simulink model "APF_CTL_VIS_Obs_2023a"  (R2023a)
settings: Solver=ode4  StartTime=0.0  StopTime=tsim  FixedStep=baseRate  RelTol=1e-6  AbsTol=1e-6
values from neighbouring files (symbols this model uses):
  A = [0 0 0 1 0 0 ... (first row only)    [CTL_NEW.m]    (also in UKF_SPOT.m = [1 0 0 dt 0 0)
  a = 25.028    [CTL_NEW.m]
  a1 = shape(1)    [Cardioid.m]    (also in Run_Initializer.m = 0.3)
  a2 = shape(2)    [Cardioid.m]    (also in Run_Initializer.m = 0.3)
  a3 = shape(3)    [Cardioid.m]    (also in Run_Initializer.m = 0.4)
  adadelta_epsilon = 1e-5    (= 1e-05)    [Run_Initializer.m]
  adadelta_gamma = 0.37    [Run_Initializer.m]
  adagrad_epsilon = 1e-8    (= 1e-08)    [Run_Initializer.m]
  adagrad_eta = 0.18    [Run_Initializer.m]
  adam_beta_1 = 0.99    [Run_Initializer.m]
  adam_beta_2 = 0.999    [Run_Initializer.m]
  adam_epsilon = 1e-2    (= 0.01)    [Run_Initializer.m]
  adam_eta = 0.0163    [Run_Initializer.m]
  adamax_beta_1 = 0.5    [Run_Initializer.m]
  adamax_beta_2 = 0.999    [Run_Initializer.m]
  adamax_eta = 0.014    [Run_Initializer.m]
  alpha_Black = 0.9    [UKF_SPOT.m]
  alpha_Blue = 0.9    [UKF_SPOT.m]
  Att_Mode = 0    [Run_Initializer.m]
  b1 = shape(4)    [Cardioid.m]    (also in Run_Initializer.m = 0.175)
  b2 = shape(5)    [Cardioid.m]    (also in Run_Initializer.m = 0.175)
  beta_Black = 2    [UKF_SPOT.m]
  beta_Blue = 20    [UKF_SPOT.m]
  Binv = inv(B)    [Run_Initializer.m]
  BLACK_end = [2, 1.4, deg2rad(368)]    [Run_Initializer.m]
  BLACK_ini = [2, 1.4, deg2rad(188), 0, 0, deg2rad(1.5)]    [Run_Initializer.m]
  BLUE_end = [1.3, 1.25, deg2rad(90)]    [Run_Initializer.m]
  BLUE_ini = [1.3, 1.25, deg2rad(270), 0, 0, deg2rad(-1.5)]    [Run_Initializer.m]
  drop_states_BLACK = BLACK_ini(1:3)    [Run_Initializer.m]
  drop_states_BLUE = BLUE_ini(1:3)    [Run_Initializer.m]
  drop_states_RED = RED_ini(1:3)    [Run_Initializer.m]
  dt = 0.01    [UKF_SPOT.m]
  end_time_black = 300    [Run_Initializer.m]
  end_time_blue = 300    [Run_Initializer.m]
  F_max = 0.22    [CTL_NEW.m]
  Gamma1_el = 0.12    [Run_Initializer.m]
  Gamma1_sh = 0.005    [Run_Initializer.m]
  Gamma1_wr = 0.025    [Run_Initializer.m]
  Gamma2_el = 5    [Run_Initializer.m]
  Gamma2_sh = 5    [Run_Initializer.m]
  Gamma2_wr = 5    [Run_Initializer.m]
  Gamma3_el = 10    [Run_Initializer.m]
  Gamma3_sh = 40    [Run_Initializer.m]
  Gamma3_wr = 40    [Run_Initializer.m]
  Gamma4_el = 0.039    [Run_Initializer.m]
  Gamma4_sh = 0.015    [Run_Initializer.m]
  Gamma4_wr = 0.029    [Run_Initializer.m]
  Gamma5_el = 800    [Run_Initializer.m]
  Gamma5_sh = 800    [Run_Initializer.m]
  Gamma5_wr = 800    [Run_Initializer.m]
  Gamma6_el = 0.000001    (= 1e-06)    [Run_Initializer.m]
  Gamma6_sh = 0.005    [Run_Initializer.m]
  Gamma6_wr = 0.02    [Run_Initializer.m]
  H = [1 0 0 0 0 0 ... (first row only)    [UKF_SPOT.m]
  home_states_BLACK = BLACK_ini(1:3)    [Run_Initializer.m]
  home_states_BLUE = BLUE_ini(1:3)    [Run_Initializer.m]
  home_states_RED = RED_ini(1:3)    [Run_Initializer.m]
  Hz = 0.01    [CTL_NEW.m]
  init_states_BLACK = BLACK_ini(1:3)    [Run_Initializer.m]
  init_states_BLUE = BLUE_ini(1:3)    [Run_Initializer.m]
  init_states_RED = RED_ini(1:3)    [Run_Initializer.m]
  J = IRED    [CTL_NEW.m]    (also in UKF_SPOT.m = 0.20184)
  k = lqr(A,B1,Q,R)    [CTL_NEW.m]
  k_1_0 = k(1,1)    [CTL_NEW.m]
  k_1_t_0 = k(3,3)    [CTL_NEW.m]
  k_2_0 = k(1,4)    [CTL_NEW.m]
  k_2_t_0 = k(3,6)    [CTL_NEW.m]
  K_a = diag([2 2 3.5])    [Run_Initializer.m]
  ka = 1    [Run_Initializer.m]
  Kd_elarm = 0.8    [Run_Initializer.m]
  Kd_sharm = 1.0    (= 1)    [Run_Initializer.m]
  Kd_t = 9.5    [CTL_NEW.m]    (also in Run_Initializer.m)
  Kd_wrarm = 0.6    [Run_Initializer.m]
  Kd_x = 28    [CTL_NEW.m]    (also in Run_Initializer.m)
  Kd_y = Kd_x    (= 28)    [CTL_NEW.m]    (also in Run_Initializer.m)
  Kp_elarm = 1.2    [Run_Initializer.m]
  Kp_sharm = 1.5    [Run_Initializer.m]
  Kp_t = 1    [CTL_NEW.m]    (also in Run_Initializer.m)
  Kp_wrarm = 2    [Run_Initializer.m]
  Kp_x = 3.5    [CTL_NEW.m]    (also in Run_Initializer.m)
  Kp_y = Kp_x    (= 3.5)    [CTL_NEW.m]    (also in Run_Initializer.m)
  kr = 2    [Run_Initializer.m]
  lambda1 = 0.4    [CTL_NEW.m]
  lambda12 = 0.4    [CTL_NEW.m]
  lambda12_t = 0.05    [CTL_NEW.m]
  lambda1_t = 0.05    [CTL_NEW.m]
  lambda2 = 0.4    [CTL_NEW.m]
  lambda2_t = 0.05    [CTL_NEW.m]
  lamda_Black = (alpha_Black^2)*(N + kappa_Black) - N    (= 15.06)    [UKF_SPOT.m]
  lamda_Blue = (alpha_Blue^2)*(N + kappa_Blue) - N    (= 6.96)    [UKF_SPOT.m]
  m = mRED    [CTL_NEW.m]    (also in UKF_SPOT.m = 11.21)
  method = 1    [UKF_SPOT.m]
  Method = 8    [Run_Initializer.m]
  momentum_eta = 0.7    [Run_Initializer.m]
  momentum_gamma = 0.7    [Run_Initializer.m]
  nesterov_eta = 0.6    [Run_Initializer.m]
  nesterov_gamma = 0.3    [Run_Initializer.m]
  Nmat = diag([1 1 1])    [Run_Initializer.m]
  p = 0.4    [CTL_NEW.m]
  P_b = diag([45 45 0])    [Run_Initializer.m]
  P_IC_Black = 0.2*eye(6)    [UKF_SPOT.m]
  P_IC_Blue = 0.2*eye(6)    [UKF_SPOT.m]
  p_t = 0.05    [CTL_NEW.m]
  psi = 1    [Run_Initializer.m]
  PWMFreq = 5    [Run_Initializer.m]
  Q = [w 0 0 0 0 0 ... (first row only)    [CTL_NEW.m]
  Q_a = diag([5, 5, 0])    [Run_Initializer.m]
  Q_b = diag([0.0125, 0.0125, 0.05])    [Run_Initializer.m]
  Q_Black = [0.0000005 0 0 0 0 0 ... (first row only)    [UKF_SPOT.m]
  Q_Blue = [0.000075 0 0 0 0 0 ... (first row only)    [UKF_SPOT.m]
  R = [r 0 0 ... (first row only)    [CTL_NEW.m]
  R_Black = [variance 0 0 ... (first row only)    [UKF_SPOT.m]
  R_Blue = [variance 0 0 ... (first row only)    [UKF_SPOT.m]
  r_hold = 0.427    [Run_Initializer.m]
  r_off = 0.165    [Run_Initializer.m]
  RED_ini = [2.7, 0.4, deg2rad(135+360), 0, 0, 0]    [Run_Initializer.m]
  Red_Rate = 0.025    [CTL_NEW.m]
  RMSprop_epsilon = 1e-8    (= 1e-08)    [Run_Initializer.m]
  RMSprop_eta = 0.025    [Run_Initializer.m]
  RMSprop_gamma = 0.9    [Run_Initializer.m]
  ... (+11 more)
undefined symbols (not defined in the file or in its folder): alpha, alpha_m, alphap, alphat, Am, b, b0, b3, baseRate, beta, Bm, c, Cm, d, DiscIntNeverNeededParam, Dm, drop_states_ARM, epsilon, F_Black_X_nominal, F_Black_Y_nominal, F_Blue_X_nominal, F_Blue_Y_nominal, F_red_X_nominal, F_red_Y_nominal, F_thrusters_BLACK, F_thrusters_BLUE, F_thrusters_RED, IBLACK, IBLUE, IDIST, IEE, IPROX, IRED, K, k1, k1t, k2, k2t, K_t, Kd_tb, Kd_tblue, Kd_tr, Kd_xb, Kd_xblue, Kd_xr, Kd_yb, Kd_yblue, Kd_yr, Kp_tb, Kp_tblue, Kp_tr, Kp_xb, Kp_xblue, Kp_xr, Kp_yb, Kp_yblue, Kp_yr, lamda ... (+34)
libraries: nvidiaSharedBlocks x10, MainLibrary x4, dspsigops x4, simulink x2, etargetslib x1
(part 15 of 15)

== matlab function APF_CTL_VIS_Obs_2023a/Phase #3: Experiment/Change RED Behavior/Sub-Phase #4/GDC/APF/GDC/Subsystem1/AdaDelta/MATLAB Function1 ==
  data: state_red input size=6; path output size=3; Eg output size=3; phi_tot_grad input size=3; Eg_old input size=3; Etheta_old input size=3; Etheta output size=3; adadelta_gamma parameter size=1; adadelta_epsilon parameter size=1
function [path, Eg, Etheta] = AdaDel(state_red, phi_tot_grad,Eg_old, Etheta_old, adadelta_gamma, adadelta_epsilon)

Eg = adadelta_gamma.*Eg_old + (1 - adadelta_gamma).*((phi_tot_grad).^2);
del_theta = (sqrt(Etheta_old + adadelta_epsilon)./sqrt(Eg + adadelta_epsilon)).*phi_tot_grad;
Etheta = adadelta_gamma.*Etheta_old + (1 - adadelta_gamma).*((del_theta).^2);

path = state_red(1:3) - del_theta;

== matlab function APF_CTL_VIS_Obs_2023a/Phase #3: Experiment/Change RED Behavior/Sub-Phase #4/GDC/APF/GDC/Subsystem1/AdaGrad/MATLAB Function1 ==
  data: state_red input; path output; phi_tot_grad input; Gt_old input; adagrad_eta parameter; Gt output; adagrad_epsilon parameter
function [path, Gt] = AdaGrad(state_red, phi_tot_grad, Gt_old,adagrad_eta, adagrad_epsilon)

Gt = Gt_old + phi_tot_grad.^2;

n = adagrad_eta./sqrt(Gt + adagrad_epsilon);

path = state_red(1:3) - n.*phi_tot_grad;

== matlab function APF_CTL_VIS_Obs_2023a/Phase #3: Experiment/Change RED Behavior/Sub-Phase #4/GDC/APF/GDC/Subsystem1/Gradient Descent/Batch ==
  data: state_red input; path output; phi_tot_grad input; batch_eta parameter
function path = gradientdescent(state_red, phi_tot_grad, batch_eta)

%Batch Gradient Descent
path = [state_red(1); state_red(2); state_red(3)] - batch_eta.*phi_tot_grad;

== matlab function APF_CTL_VIS_Obs_2023a/Phase #3: Experiment/Change RED Behavior/Sub-Phase #4/GDC/APF/GDC/Subsystem1/AdaMax/MATLAB Function1 ==
  data: state_red input; path output; phi_tot_grad input; m_old input; m output; u_old input; time input; u_t output; adamax_beta_1 parameter; adamax_beta_2 parameter; adamax_eta parameter
function [path, m, u_t] = AdaMax(state_red, phi_tot_grad,m_old, u_old, time, adamax_beta_1, adamax_beta_2, adamax_eta)

t = time/0.1;
m = adamax_beta_1.*m_old + (1 - adamax_beta_1).*phi_tot_grad;
%v = adamax_beta_2.*v_old + (1 - adamax_beta_2).*norm(phi_tot_grad,"inf");

m_h = m./(1 - (adamax_beta_1)^(t + 1));
u_t = max(adamax_beta_2.*u_old, abs(phi_tot_grad));

path = state_red(1:3) - (adamax_eta./u_t).*m_h;

== matlab function APF_CTL_VIS_Obs_2023a/Phase #4: Return Home/Change BLACK Behavior/Hough Control/MATLAB Function2 ==
  data: Oy output; z input; Ox output
function [Oy, Ox]   = C3( z )
%C3 gives the rotation matrix about the z-axis for an angle 'z'
%   z - the angle about the z-axis which you rotate
%   A - the rotation matrix

Ox = [cos(z) sin(z); -sin(z) cos(z)]*[1;0];
Oy = [cos(z) sin(z); -sin(z) cos(z)]*[0;1];
end

== matlab function APF_CTL_VIS_Obs_2023a/Phase #4: Return Home/Change BLACK Behavior/Hough Control/MATLAB Function3 ==
  data: z input; Ox output
function Ox    = C3( z )
%C3 gives the rotation matrix about the z-axis for an angle 'z'
%   z - the angle about the z-axis which you rotate
%   A - the rotation matrix

Ox = [cos(z) sin(z); -sin(z) cos(z)]*[1;0];
end

== matlab function APF_CTL_VIS_Obs_2023a/Phase #4: Return Home/Change BLACK Behavior/Hough Control/MATLAB Function4 ==
  data: Oy input; e_out output; e_in input
function e_out = fcn(Oy, e_in)

a = sign(Oy'*e_in);
e_out = -a*norm(e_in);

== matlab function APF_CTL_VIS_Obs_2023a/Phase #3: Experiment/Change RED Behavior/Sub-Phase #4/GDC/APF/GDC/Subsystem1/Adam/MATLAB Function1 ==
  data: state_red input; path output; phi_tot_grad input; m_old input; m output; v_old input; time input; v output; adam_beta_1 parameter; adam_beta_2 parameter; adam_eta parameter; adam_epsilon parameter
function [path, m, v] = Adam(state_red, phi_tot_grad,m_old, v_old, time, adam_beta_1, adam_beta_2, adam_eta, adam_epsilon)

m = adam_beta_1.*m_old + (1 - adam_beta_1).*phi_tot_grad;
v = adam_beta_2.*v_old + (1 - adam_beta_2).*(phi_tot_grad).^2;

m_h = m./(1 - (adam_beta_1)^(time/0.1 + 1));
v_h = v./(1 - (adam_beta_2)^(time/0.1 + 1));

path = state_red(1:3) - (adam_eta./(sqrt(v_h) + adam_epsilon)).*m_h;

== matlab function APF_CTL_VIS_Obs_2023a/Phase #3: Experiment/Change RED Behavior/Sub-Phase #4/GDC/APF/GDC/Subsystem1/Nesterov/MATLAB Function1 ==
  data: state_red input; path output; v_prev input; shape parameter; ka parameter; kr parameter; Q_a parameter; Q_b parameter; P_b parameter; r_hold parameter; Binv parameter; K_a parameter; psi parameter; sigma parameter; r_off parameter; Nmat parameter; nesterov_gamma parameter; v output; state_black input; state_blue input; nesterov_eta parameter; isBlue input
function [path, v] = nesterov(state_red, v_prev, shape, ka, kr, Q_a, Q_b, P_b, r_hold, Binv, K_a, psi, sigma, r_off, Nmat, nesterov_gamma, state_black, state_blue, nesterov_eta,isBlue)
%Nesterov Accelerated Gradient

state_red_est = state_red + nesterov_gamma.*[v_prev(1); v_prev(2); v_prev(3); 0; 0; 0];
[~,phi_tot_grad,~,~] = APF_func_Maybe_Obstacle(state_red_est,state_black,state_blue,shape,ka,kr,Q_a,Q_b,P_b,r_hold,Binv,K_a,psi,sigma,r_off,Nmat,isBlue); %calculates the gradient if 

v = -nesterov_gamma*v_prev-nesterov_eta.*phi_tot_grad;
path = [state_red(1); state_red(2); state_red(3)] + v;

== matlab function APF_CTL_VIS_Obs_2023a/Phase #3: Experiment/Change BLUE Behavior/Sub-Phase #1/BLUE_Rz Desired/Wrap/MATLAB Function ==
  data: u input; wrappedAngle output
function wrappedAngle = wrapAngle(u)

wrappedAngle = atan2(sin(u),cos(u));

end

== matlab function APF_CTL_VIS_Obs_2023a/Phase #3: Experiment/Change BLACK Behavior/Sub-Phase #4/Hough Control/MATLAB Function4 ==
  data: Oy input; e_out output; e_in input
function e_out = fcn(Oy, e_in)

a = sign(Oy'*e_in);
e_out = -a*norm(e_in);

== matlab function APF_CTL_VIS_Obs_2023a/Phase #4: Return Home/Change BLUE Behavior/Hough Control/MATLAB Function2 ==
  data: Oy output; z input; Ox output
function [Oy, Ox]   = C3( z )
%C3 gives the rotation matrix about the z-axis for an angle 'z'
%   z - the angle about the z-axis which you rotate
%   A - the rotation matrix

Ox = [cos(z) sin(z); -sin(z) cos(z)]*[1;0];
Oy = [cos(z) sin(z); -sin(z) cos(z)]*[0;1];
end

== matlab function APF_CTL_VIS_Obs_2023a/Phase #4: Return Home/Change BLUE Behavior/Hough Control/MATLAB Function3 ==
  data: z input; Ox output
function Ox    = C3( z )
%C3 gives the rotation matrix about the z-axis for an angle 'z'
%   z - the angle about the z-axis which you rotate
%   A - the rotation matrix

Ox = [cos(z) sin(z); -sin(z) cos(z)]*[1;0];
end

== matlab function APF_CTL_VIS_Obs_2023a/Phase #4: Return Home/Change BLUE Behavior/Hough Control/MATLAB Function4 ==
  data: Oy input; e_out output; e_in input
function e_out = fcn(Oy, e_in)

a = sign(Oy'*e_in);
e_out = -a*norm(e_in);

== matlab function APF_CTL_VIS_Obs_2023a/Phase #4: Return Home/Change RED Behavior/Hough Control/MATLAB Function2 ==
  data: Oy output; z input; Ox output
function [Oy, Ox]   = C3( z )
%C3 gives the rotation matrix about the z-axis for an angle 'z'
%   z - the angle about the z-axis which you rotate
%   A - the rotation matrix

Ox = [cos(z) sin(z); -sin(z) cos(z)]*[1;0];
Oy = [cos(z) sin(z); -sin(z) cos(z)]*[0;1];
end

== matlab function APF_CTL_VIS_Obs_2023a/Phase #4: Return Home/Change RED Behavior/Hough Control/MATLAB Function3 ==
  data: z input; Ox output
function Ox    = C3( z )
%C3 gives the rotation matrix about the z-axis for an angle 'z'
%   z - the angle about the z-axis which you rotate
%   A - the rotation matrix

Ox = [cos(z) sin(z); -sin(z) cos(z)]*[1;0];
end

== matlab function APF_CTL_VIS_Obs_2023a/Phase #4: Return Home/Change RED Behavior/Hough Control/MATLAB Function4 ==
  data: Oy input; e_out output; e_in input
function e_out = fcn(Oy, e_in)

a = sign(Oy'*e_in);
e_out = -a*norm(e_in);

== matlab function APF_CTL_VIS_Obs_2023a/Thruster Control Code/Change RED Behavior/Calculate Thruster ON//OFF/MATLAB Function ==
  data: H output; thruster_dist2CG_RED parameter; F_thrusters_RED parameter; theta_1 input; theta_2 input; theta_3 input; mRED parameter; mPROX parameter; mDIST parameter; mEE parameter; Phi parameter; b0 parameter; a1 parameter; b1 parameter; a2 parameter; b2 parameter; a3 parameter; b3 parameter
function H   = MakeHWithArm(thruster_dist2CG_RED,F_thrusters_RED, theta_1, theta_2, theta_3, mRED, mPROX, mDIST, mEE, Phi, b0, a1, b1, a2, b2, a3, b3)
    
    link1_com_x = b0*cos(Phi) + a1*cos(pi/2 + theta_1);
    link1_com_y = b0*sin(Phi) + a1*sin(pi/2 + theta_1);
    
    link2_com_x = link1_com_x + b1*cos(pi/2 + theta_1) + a2*cos(pi/2 + theta_1 + theta_2);
    link2_com_y = link1_com_y + b1*sin(pi/2 + theta_1) + a2*sin(pi/2 + theta_1 + theta_2);
    
    link3_com_x = link2_com_x + b2*cos(pi/2 + theta_1 + theta_2) + a3*cos(pi/2 + theta_1 + theta_2 + theta_3);
    link3_com_y = link2_com_y + b2*sin(pi/2 + theta_1 + theta_2) + a3*sin(pi/2 + theta_1 + theta_2 + theta_3);
    
    delta_com_due_to_arm_x = (mPROX*link1_com_x + mDIST*link2_com_x + mEE*link3_com_x)/(mRED + mPROX + mDIST + mEE)*1000; % [mm]
    delta_com_due_to_arm_y = (mPROX*link1_com_y + mDIST*link2_com_y + mEE*link3_com_y)/(mRED + mPROX + mDIST + mEE)*1000; % [mm]
    
    adjusted_thruster_dist2CG_RED = [thruster_dist2CG_RED(1)-delta_com_due_to_arm_y;
                                     thruster_dist2CG_RED(2)-delta_com_due_to_arm_y;
                                     thruster_dist2CG_RED(3)-delta_com_due_to_arm_x;
                                     thruster_dist2CG_RED(4)-delta_com_due_to_arm_x;
                                     thruster_dist2CG_RED(5)+delta_com_due_to_arm_y;
                                     thruster_dist2CG_RED(6)+delta_com_due_to_arm_y;
                                     thruster_dist2CG_RED(7)+delta_com_due_to_arm_x;
                                     thruster_dist2CG_RED(8)+delta_com_due_to_arm_x];
                                     
    
    
    Vec1 = [ -1
             -1
              0 
              0
              1
              1
              0
              0 ];
          
    Vec2 = [  0
              0
              1
              1
              0
              0
             -1
             -1 ];
         
    Vec3 = adjusted_thruster_dist2CG_RED./1000;
    
    Mat1 = [Vec1, Vec2, Vec3]';
    
    Mat2 = diag((F_thrusters_RED./2));
    
    H    = Mat1*Mat2;

end

== matlab function APF_CTL_VIS_Obs_2023a/Phase #3: Experiment/Change BLUE Behavior/Sub-Phase #2 /BLUE_Rz Desired/Wrap/MATLAB Function ==
  data: u input; wrappedAngle output
function wrappedAngle = wrapAngle(u)

wrappedAngle = atan2(sin(u),cos(u));

end

== matlab function APF_CTL_VIS_Obs_2023a/Thruster Control Code/Change BLACK Behavior/Calculate Thruster ON//OFF/MATLAB Function3 ==
  data: H output; thruster_dist2CG_BLACK parameter; F_Black_X_nominal parameter; thrust_decay_factor input; F_Black_Y_nominal parameter
function H   = MakeHWithDecay(thruster_dist2CG_BLACK,F_Black_X_nominal, thrust_decay_factor, F_Black_Y_nominal)


adjusted_thruster_dist2CG_BLACK = [thruster_dist2CG_BLACK(1);
                                 thruster_dist2CG_BLACK(2);
                                 thruster_dist2CG_BLACK(3);
                                 thruster_dist2CG_BLACK(4);
                                 thruster_dist2CG_BLACK(5);
                                 thruster_dist2CG_BLACK(6);
                                 thruster_dist2CG_BLACK(7);
                                 thruster_dist2CG_BLACK(8)];
                                 


Vec1 = [ -1
         -1
          0 
          0
          1
          1
          0
          0 ];
      
Vec2 = [  0
          0
          1
          1
          0
          0
         -1
         -1 ];
     
Vec3 = adjusted_thruster_dist2CG_BLACK./1000;

Mat1 = [Vec1, Vec2, Vec3]';

F_thrusters_BLACK = [F_Black_X_nominal*thrust_decay_factor; F_Black_X_nominal*thrust_decay_factor; F_Black_Y_nominal*thrust_decay_factor; F_Black_Y_nominal*thrust_decay_factor; F_Black_X_nominal*thrust_decay_factor; F_Black_X_nominal*thrust_decay_factor; F_Black_Y_nominal*thrust_decay_factor; F_Black_Y_nominal*thrust_decay_factor];

Mat2 = diag((F_thrusters_BLACK));

H    = Mat1*Mat2;

end

== matlab function APF_CTL_VIS_Obs_2023a/Thruster Control Code/Change RED Behavior/Calculate Thruster ON//OFF/MATLAB Function2 ==
  data: ThrustPer_Final output; ThrustPer input; PWMFreq parameter
function ThrustPer_Final  = ThrusterSat(ThrustPer, PWMFreq)

    ValveTime       = 0.007;
    TControl        = 1/PWMFreq;

    ThrustPer_Final = zeros(8,1);
    
    if max(ThrustPer) > 1
        ThrustPer_Sat = ThrustPer/max(ThrustPer);
    else
        ThrustPer_Sat = ThrustPer;
    end
    
    for i = 1:8
        if ThrustPer_Sat(i) > ValveTime/TControl 
            ThrustPer_Final(i) = ThrustPer_Sat(i);
        else
            ThrustPer_Final(i) = 0;
        end
    end


end

== matlab function APF_CTL_VIS_Obs_2023a/Thruster Control Code/Change RED Behavior/Calculate Thruster ON//OFF/Rotate Forces to Inertial/Create Rotation Matrix ==
  data: Rz input; C_Ib output
function C_Ib = RotateFrame(Rz)

C_bI = [  cos(Rz) sin(Rz)
         -sin(Rz) cos(Rz) ];

C_Ib = inv(C_bI);

end

== matlab function APF_CTL_VIS_Obs_2023a/Phase #3: Experiment/Change BLACK Behavior/Sub-Phase #2 /BLACK_Rz Desired/Wrap1/MATLAB Function ==
  data: u input; wrappedAngle output
function wrappedAngle = wrapAngle(u)

wrappedAngle = atan2(sin(u),cos(u));

end

== matlab function APF_CTL_VIS_Obs_2023a/Phase #3: Experiment/Change RED Behavior/Sub-Phase #1/MATLAB Function ==
  data: t input; x output; xLength parameter
function x = fcn(t, xLength)

x = 0.9*cos((0.03490659)*t) + xLength/2;

end

== matlab function APF_CTL_VIS_Obs_2023a/Phase #3: Experiment/Change RED Behavior/Sub-Phase #4/GDC/APF/GDC/Subsystem1/RMSProp/MATLAB Function1 ==
  data: state_red input; path output; phi_tot_grad input; Eg_old input; Eg output; RMSprop_eta parameter; RMSprop_gamma parameter; RMSprop_epsilon parameter
function [path, Eg] = RMSProp(state_red, phi_tot_grad, Eg_old, RMSprop_eta, RMSprop_gamma, RMSprop_epsilon)

Eg = RMSprop_gamma.*Eg_old + (1 - RMSprop_gamma).*((phi_tot_grad).^2);

n = RMSprop_eta./sqrt(Eg + RMSprop_epsilon);

path = state_red(1:3) - n.*phi_tot_grad;

== matlab function APF_CTL_VIS_Obs_2023a/Simulate Plant Dynamics/RED and ARM Dynamics/RED + ARM/RED + ARM Dynamics/Dynamics Model ==
  data: xdot output; x input; InertiaS input; CoriolisS input; u input; Gamma1_sh parameter; Gamma2_sh parameter; Gamma3_sh parameter; Gamma5_sh parameter; Gamma4_sh parameter; Gamma6_sh parameter; Gamma1_el parameter; Gamma2_el parameter; Gamma3_el parameter; Gamma5_el parameter; Gamma4_el parameter; Gamma6_el parameter; Gamma1_wr parameter; Gamma2_wr parameter; Gamma3_wr parameter; Gamma5_wr parameter; Gamma4_wr parameter; Gamma6_wr parameter
function xdot  = DynamicsModel(x, InertiaS, CoriolisS, u,...
    Gamma1_sh, Gamma2_sh, Gamma3_sh, Gamma5_sh, Gamma4_sh, Gamma6_sh,...
    Gamma1_el, Gamma2_el, Gamma3_el, Gamma5_el, Gamma4_el, Gamma6_el,...
    Gamma1_wr, Gamma2_wr, Gamma3_wr, Gamma5_wr, Gamma4_wr, Gamma6_wr)


    fqdot1 = Gamma1_sh*(tanh(Gamma2_sh*x(10)) - tanh(Gamma3_sh*x(10))) + Gamma4_sh*tanh(Gamma5_sh*x(10)) + Gamma6_sh*x(10);

    fqdot2 = Gamma1_el*(tanh(Gamma2_el*x(11)) - tanh(Gamma3_el*x(11))) + Gamma4_el*tanh(Gamma5_el*x(11)) + Gamma6_el*x(11);

    fqdot3 = Gamma1_wr*(tanh(Gamma2_wr*x(12)) - tanh(Gamma3_wr*x(12))) + Gamma4_wr*tanh(Gamma5_wr*x(12)) + Gamma6_wr*x(12);
    
    q_ddot = pinv(InertiaS)*(u - CoriolisS*x(7:12) - [0;0;0;fqdot1;fqdot2;fqdot3]);
    
    xdot   = [ x(7:12)
               q_ddot   ];
           
end

== matlab function APF_CTL_VIS_Obs_2023a/Phase #3: Experiment/Change BLUE Behavior/Sub-Phase #3 /BLUE_Rz Desired/Wrap/MATLAB Function ==
  data: u input; wrappedAngle output
function wrappedAngle = wrapAngle(u)

wrappedAngle = atan2(sin(u),cos(u));

end

== matlab function APF_CTL_VIS_Obs_2023a/Phase #3: Experiment/Change RED Behavior/Sub-Phase #4/CTL/If Action Subsystem/Homo/MATLAB Function2 ==
  data: q1 input; u output; k1 parameter; alphap parameter
function u = fcn(q1,k1, alphap)

u = k1*sign(q1)*(abs(q1)^(alphap/(2 - alphap)));

== matlab function APF_CTL_VIS_Obs_2023a/Phase #3: Experiment/Change RED Behavior/Sub-Phase #1/MATLAB Function1 ==
  data: t input; y output; yLength parameter
function y = fcn(t, yLength)

y = 0.85*sin((0.03490659)*t) + yLength/2;

end

== matlab function APF_CTL_VIS_Obs_2023a/Phase #3: Experiment/Change RED Behavior/Sub-Phase #2 /Hough Control/MATLAB Function2 ==
  data: Oy output; z input; Ox output
function [Oy, Ox]   = C3( z )
%C3 gives the rotation matrix about the z-axis for an angle 'z'
%   z - the angle about the z-axis which you rotate
%   A - the rotation matrix

Ox = [cos(z) sin(z); -sin(z) cos(z)]*[1;0];
Oy = [cos(z) sin(z); -sin(z) cos(z)]*[0;1];
end

== matlab function APF_CTL_VIS_Obs_2023a/Phase #3: Experiment/Change RED Behavior/Sub-Phase #2 /Hough Control/MATLAB Function3 ==
  data: z input; Ox output
function Ox    = C3( z )
%C3 gives the rotation matrix about the z-axis for an angle 'z'
%   z - the angle about the z-axis which you rotate
%   A - the rotation matrix

Ox = [cos(z) sin(z); -sin(z) cos(z)]*[1;0];
end

== matlab function APF_CTL_VIS_Obs_2023a/Phase #3: Experiment/Change BLACK Behavior/Sub-Phase #2 /Hough Control/MATLAB Function2 ==
  data: Oy output; z input; Ox output
function [Oy, Ox]   = C3( z )
%C3 gives the rotation matrix about the z-axis for an angle 'z'
%   z - the angle about the z-axis which you rotate
%   A - the rotation matrix

Ox = [cos(z) sin(z); -sin(z) cos(z)]*[1;0];
Oy = [cos(z) sin(z); -sin(z) cos(z)]*[0;1];
end

== matlab function APF_CTL_VIS_Obs_2023a/Phase #3: Experiment/Change RED Behavior/Sub-Phase #2 /Hough Control/MATLAB Function4 ==
  data: Oy input; e_out output; e_in input
function e_out = fcn(Oy, e_in)

a = sign(Oy'*e_in);
e_out = -a*norm(e_in);

== matlab function APF_CTL_VIS_Obs_2023a/Thruster Control Code/Change RED Behavior/Calculate Thruster ON//OFF/MATLAB Function3 ==
  data: H output; thruster_dist2CG_RED parameter; F_thrusters_RED parameter
function H = MakeH(thruster_dist2CG_RED,F_thrusters_RED)

Vec1 = [ -1
         -1
          0 
          0
          1
          1
          0
          0 ];
      
Vec2 = [  0
          0
          1
          1
          0
          0
         -1
         -1 ];
     
Vec3 = thruster_dist2CG_RED./1000;

Mat1 = [Vec1, Vec2, Vec3]';

Mat2 = diag((F_thrusters_RED));

H    = Mat1*Mat2;

end

== matlab function APF_CTL_VIS_Obs_2023a/Phase #3: Experiment/Change BLUE Behavior/Sub-Phase #4/BLUE_Rz Desired/Wrap/MATLAB Function ==
  data: u input; wrappedAngle output
function wrappedAngle = wrapAngle(u)

wrappedAngle = atan2(sin(u),cos(u));

end

== matlab function APF_CTL_VIS_Obs_2023a/Thruster Control Code/Change RED Behavior/Calculate Thruster ON//OFF/MATLAB Function4 ==
  data: H output; thruster_dist2CG_RED parameter; F_red_X_nominal parameter; theta_1 input; theta_2 input; theta_3 input; mRED parameter; thrust_decay_factor input; F_red_Y_nominal parameter; mPROX parameter; mDIST parameter; mEE parameter; Phi parameter; b0 parameter; a1 parameter; b1 parameter; a2 parameter; b2 parameter; a3 parameter; b3 parameter
function H   = MakeH(thruster_dist2CG_RED,F_red_X_nominal, theta_1, theta_2, theta_3, mRED, thrust_decay_factor, F_red_Y_nominal, mPROX, mDIST, mEE, Phi, b0, a1, b1, a2, b2, a3, b3)
    
    link1_com_x = b0*cos(Phi) + a1*cos(pi/2 + theta_1);
    link1_com_y = b0*sin(Phi) + a1*sin(pi/2 + theta_1);
    
    link2_com_x = link1_com_x + b1*cos(pi/2 + theta_1) + a2*cos(pi/2 + theta_1 + theta_2);
    link2_com_y = link1_com_y + b1*sin(pi/2 + theta_1) + a2*sin(pi/2 + theta_1 + theta_2);
    
    link3_com_x = link2_com_x + b2*cos(pi/2 + theta_1 + theta_2) + a3*cos(pi/2 + theta_1 + theta_2 + theta_3);
    link3_com_y = link2_com_y + b2*sin(pi/2 + theta_1 + theta_2) + a3*sin(pi/2 + theta_1 + theta_2 + theta_3);
    
    delta_com_due_to_arm_x = (mPROX*link1_com_x + mDIST*link2_com_x + mEE*link3_com_x)/(mRED + mPROX + mDIST + mEE)*1000; % [mm]
    delta_com_due_to_arm_y = (mPROX*link1_com_y + mDIST*link2_com_y + mEE*link3_com_y)/(mRED + mPROX + mDIST + mEE)*1000; % [mm]
    
    adjusted_thruster_dist2CG_RED = [thruster_dist2CG_RED(1)-delta_com_due_to_arm_y;
                                     thruster_dist2CG_RED(2)-delta_com_due_to_arm_y;
                                     thruster_dist2CG_RED(3)-delta_com_due_to_arm_x;
                                     thruster_dist2CG_RED(4)-delta_com_due_to_arm_x;
                                     thruster_dist2CG_RED(5)+delta_com_due_to_arm_y;
                                     thruster_dist2CG_RED(6)+delta_com_due_to_arm_y;
                                     thruster_dist2CG_RED(7)+delta_com_due_to_arm_x;
                                     thruster_dist2CG_RED(8)+delta_com_due_to_arm_x];
                                     
    
    
    Vec1 = [ -1
             -1
              0 
              0
              1
              1
              0
              0 ];
          
    Vec2 = [  0
              0
              1
              1
              0
              0
             -1
             -1 ];
         
    Vec3 = adjusted_thruster_dist2CG_RED./1000;
    
    Mat1 = [Vec1, Vec2, Vec3]';
    
    F_thrusters_RED = [F_red_X_nominal*thrust_decay_factor; F_red_X_nominal*thrust_decay_factor; F_red_Y_nominal*thrust_decay_factor; F_red_Y_nominal*thrust_decay_factor; F_red_X_nominal*thrust_decay_factor; F_red_X_nominal*thrust_decay_factor; F_red_Y_nominal*thrust_decay_factor; F_red_Y_nominal*thrust_decay_factor];
    
    Mat2 = diag((F_thrusters_RED));
    
    H    = Mat1*Mat2;

end

== matlab function APF_CTL_VIS_Obs_2023a/Thruster Control Code/Change RED Behavior/Calculate Thruster ON//OFF/MATLAB Function5 ==
  data: thrust_decay_factor output; PWMs input; thruster_count_threshold parameter; count output
function [thrust_decay_factor, count]  = check_thrust_decay(PWMs,thruster_count_threshold)

% normalize PWMs
if max(PWMs) > 1
    PWMs = PWMs/max(PWMs);
end

count = sum(PWMs > thruster_count_threshold);

positives_only = max(PWMs,0);
sum_of_duty_cycles = sum(positives_only);

average_duty_cycle_per_thruster = sum_of_duty_cycles/count;

% Look up the thrust decay for this average duty cycle
if (average_duty_cycle_per_thruster < 0.3) || (count == 0)
    thrust_decay_factor = 1;
else
    thrust_decay_factor = max(0.6 - 2*average_duty_cycle_per_thruster + 1, 0.5);   
end

== matlab function APF_CTL_VIS_Obs_2023a/Thruster Control Code/Change RED Behavior/Calculate Thruster ON//OFF/MATLAB Function6 ==
  data: H output; thruster_dist2CG_RED parameter; F_red_X_nominal parameter; theta_1 input; theta_2 input; theta_3 input; mRED parameter; thrust_decay_factor input; F_red_Y_nominal parameter; mPROX parameter; mDIST parameter; mEE parameter; Phi parameter; b0 parameter; a1 parameter; b1 parameter; a2 parameter; b2 parameter; a3 parameter; b3 parameter
function H   = MakeHWithArmAndDecay(thruster_dist2CG_RED,F_red_X_nominal, theta_1, theta_2, theta_3,  mRED, thrust_decay_factor, F_red_Y_nominal, mPROX, mDIST, mEE, Phi, b0, a1, b1, a2, b2, a3, b3)
    
    link1_com_x = b0*cos(Phi) + a1*cos(pi/2 + theta_1);
    link1_com_y = b0*sin(Phi) + a1*sin(pi/2 + theta_1);
    
    link2_com_x = link1_com_x + b1*cos(pi/2 + theta_1) + a2*cos(pi/2 + theta_1 + theta_2);
    link2_com_y = link1_com_y + b1*sin(pi/2 + theta_1) + a2*sin(pi/2 + theta_1 + theta_2);
    
    link3_com_x = link2_com_x + b2*cos(pi/2 + theta_1 + theta_2) + a3*cos(pi/2 + theta_1 + theta_2 + theta_3);
    link3_com_y = link2_com_y + b2*sin(pi/2 + theta_1 + theta_2) + a3*sin(pi/2 + theta_1 + theta_2 + theta_3);
    
    delta_com_due_to_arm_x = (mPROX*link1_com_x + mDIST*link2_com_x + mEE*link3_com_x)/(mRED + mPROX + mDIST + mEE)*1000; % [mm]
    delta_com_due_to_arm_y = (mPROX*link1_com_y + mDIST*link2_com_y + mEE*link3_com_y)/(mRED + mPROX + mDIST + mEE)*1000; % [mm]
    
    adjusted_thruster_dist2CG_RED = [thruster_dist2CG_RED(1)-delta_com_due_to_arm_y;
                                     thruster_dist2CG_RED(2)-delta_com_due_to_arm_y;
                                     thruster_dist2CG_RED(3)-delta_com_due_to_arm_x;
                                     thruster_dist2CG_RED(4)-delta_com_due_to_arm_x;
                                     thruster_dist2CG_RED(5)+delta_com_due_to_arm_y;
                                     thruster_dist2CG_RED(6)+delta_com_due_to_arm_y;
                                     thruster_dist2CG_RED(7)+delta_com_due_to_arm_x;
                                     thruster_dist2CG_RED(8)+delta_com_due_to_arm_x];
                                 
    
    
    Vec1 = [ -1
             -1
              0 
              0
              1
              1
              0
              0 ];
          
    Vec2 = [  0
              0
              1
              1
              0
              0
             -1
             -1 ];
         
    Vec3 = adjusted_thruster_dist2CG_RED./1000;
    
    Mat1 = [Vec1, Vec2, Vec3]';
    
    F_thrusters_RED = [F_red_X_nominal*thrust_decay_factor; F_red_X_nominal*thrust_decay_factor; F_red_Y_nominal*thrust_decay_factor; F_red_Y_nominal*thrust_decay_factor; F_red_X_nominal*thrust_decay_factor; F_red_X_nominal*thrust_decay_factor; F_red_Y_nominal*thrust_decay_factor; F_red_Y_nominal*thrust_decay_factor];
    
    Mat2 = diag((F_thrusters_RED./2));
    
    H    = Mat1*Mat2;

end

== matlab function APF_CTL_VIS_Obs_2023a/Phase #3: Experiment/Change BLACK Behavior/Sub-Phase #2 /Hough Control/MATLAB Function3 ==
  data: z input; Ox output
function Ox    = C3( z )
%C3 gives the rotation matrix about the z-axis for an angle 'z'
%   z - the angle about the z-axis which you rotate
%   A - the rotation matrix

Ox = [cos(z) sin(z); -sin(z) cos(z)]*[1;0];
end

== matlab function APF_CTL_VIS_Obs_2023a/Phase #5: Hold Home/Change BLACK Behavior/Hough Control/MATLAB Function2 ==
  data: Oy output; z input; Ox output
function [Oy, Ox]   = C3( z )
%C3 gives the rotation matrix about the z-axis for an angle 'z'
%   z - the angle about the z-axis which you rotate
%   A - the rotation matrix

Ox = [cos(z) sin(z); -sin(z) cos(z)]*[1;0];
Oy = [cos(z) sin(z); -sin(z) cos(z)]*[0;1];
end

== matlab function APF_CTL_VIS_Obs_2023a/Phase #3: Experiment/Change BLACK Behavior/Sub-Phase #2 /Hough Control/MATLAB Function4 ==
  data: Oy input; e_out output; e_in input
function e_out = fcn(Oy, e_in)

a = sign(Oy'*e_in);
e_out = -a*norm(e_in);
